simulink library "SLUGS_Library"  (Simulink 6.6)
values from neighbouring files (symbols this model uses):
  T = 0.01    [initGPS.m]    (also in mcuInit.m)
undefined symbols (not defined in the file or in its folder): apSampleTime, bankCommandLimit, daLimit, deLimit, DiscIntNeverNeededParam, drLimit, dtLimit, gaind, getWP, heightErrorLimit, mass, Ndelay, param, pitchCommandLimit, pitchErrorLimit, polesd, rollControlLimit, SampleT, Ts, u1, Xpoints, y1, yawDamperLimit, yo, Ypoints, zerosd, Zpoints
libraries: SLUGS_Library x51, simulink x32, dsPICdrivers x13, aerolibutil x2, aerolibconvert2 x1
(part 1 of 2)
settings Model: Creator=Administrator  LastModifiedBy=Elkaim

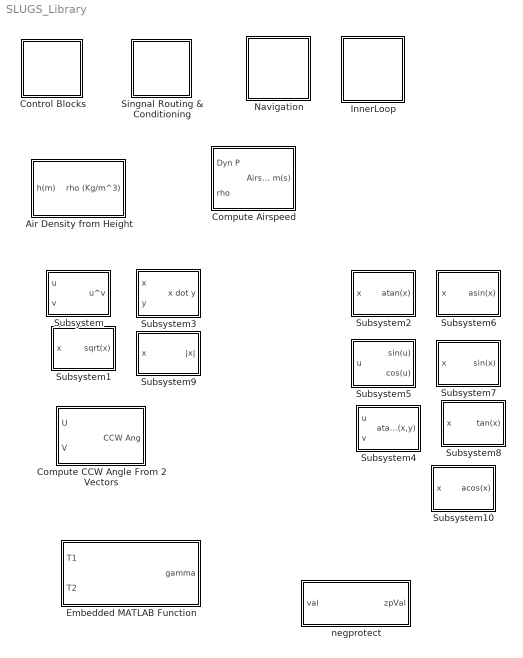
== system SLUGS_Library ==
  Air Density from Height : Subsystem  AncestorBlock=SLUGS_Library/Air Density from Height
  Compute Airspeed : Subsystem  AncestorBlock=SLUGS_Library/Compute Airspeed
  Compute CCW Angle From 2 Vectors : Subsystem
  Control Blocks : Subsystem
  Embedded MATLAB Function : Stateflow chart
  InnerLoop : Subsystem
  Navigation : Subsystem
  Singnal Routing & Conditioning : Subsystem
  Subsystem : Subsystem  AncestorBlock=SLUGS_Library/Air Density from Height/Subsystem
  Subsystem1 : Subsystem  AncestorBlock=SLUGS_Library/Compute Airspeed/Subsystem
  Subsystem10 : Subsystem
  Subsystem2 : Subsystem
  Subsystem3 : Subsystem
  Subsystem4 : Subsystem  AncestorBlock=SLUGS_Library/Air Density from Height/Subsystem
  Subsystem5 : Subsystem
  Subsystem6 : Subsystem  AncestorBlock=SLUGS_Library/Subsystem2
  Subsystem7 : Subsystem  AncestorBlock=SLUGS_Library/Subsystem2
  Subsystem8 : Subsystem
  Subsystem9 : Subsystem
  negprotect : Stateflow chart

== system SLUGS_Library/Air Density from Height ==
  h(m) : Inport
  Add : Sum  Inputs=+-  OutScaling=2^-10
  Constant : Constant  OutDataTypeMode=single
  Constant 2 from Model : Constant  Value=4.255876  OutDataTypeMode=single
  Constant from Model : Constant  Value=145442  OutDataTypeMode=single
  Divide : Product  Inputs=*/  OutScaling=2^-10
  Divide1 : Product  OutScaling=2^-10
  Length Conversion : aerolibconvert2/Length Conversion  SystemSampleTime=-1  IU=m  OU=ft
  Rho_0 (Kg/m^3) : Constant  Value=1.225  OutDataTypeMode=single
  Subsystem : SLUGS_Library/Subsystem  SystemSampleTime=-1
  rho (Kg/m^3) : Outport
  wires:
  Subsystem/1 -> Divide1/1
  Constant 2 from Model/1 -> Subsystem/2
  Add/1 -> Subsystem/1
  Length Conversion/1 -> Divide/1
  Divide1/1 -> rho (Kg/m^3)/1
  Rho_0 (Kg/m^3)/1 -> Divide1/2
  Constant from Model/1 -> Divide/2
  h(m)/1 -> Length Conversion/1
  Divide/1 -> Add/2
  Constant/1 -> Add/1

== system SLUGS_Library/Compute Airspeed ==
  Dyn P : Inport
  rho : Inport  Port=2
  Divide2 : Product  Inputs=**/  OutScaling=2^-10
  Subsystem1 : SLUGS_Library/Subsystem1  SystemSampleTime=-1
  "[ 0.01 50000]" : Saturate  UpperLimit=50000  LowerLimit=0.01
  a : Constant  Value=2  OutDataTypeMode=single
  Airspeed m(s) : Outport
  wires:
  Divide2/1 -> Subsystem1/1
  Subsystem1/1 -> Airspeed m(s)/1
  a/1 -> Divide2/1
  Dyn P/1 -> Divide2/2
  rho/1 -> "[ 0.01 50000]"/1
  "[ 0.01 50000]"/1 -> Divide2/3

== system SLUGS_Library/Compute CCW Angle From 2 Vectors ==
  U : Inport
  V : Inport  Port=2
  Add : Sum  Inputs=+-  OutScaling=2^-10
  Embedded MATLAB Function1 : Stateflow chart
  Selector : Selector  IndexOptions=Index vector (dialog)  Indices=[1]  OutputSizes=1  InputPortWidth=3
  Selector1 : Selector  IndexOptions=Index vector (dialog)  Indices=[1]  OutputSizes=1  InputPortWidth=3
  Selector2 : Selector  IndexOptions=Index vector (dialog)  Indices=[2]  OutputSizes=1  InputPortWidth=3
  Selector3 : Selector  IndexOptions=Index vector (dialog)  Indices=[2]  OutputSizes=1  InputPortWidth=3
  Subsystem1 : SLUGS_Library/Subsystem4  SystemSampleTime=-1
  Subsystem4 : SLUGS_Library/Subsystem4  SystemSampleTime=-1
  CCW Ang : Outport
  wires:
  Embedded MATLAB Function1/1(angle) -> CCW Ang/1
  V/1 -> Selector1/1, Selector2/1
  U/1 -> Selector/1, Selector3/1
  Add/1 -> Embedded MATLAB Function1/1(rawAngle)
  Subsystem1/1 -> Add/2
  Subsystem4/1 -> Add/1
  Selector1/1 -> Subsystem1/2
  Selector2/1 -> Subsystem1/1
  Selector/1 -> Subsystem4/2
  Selector3/1 -> Subsystem4/1

== system SLUGS_Library/Control Blocks ==
  PD Controller  Internal Derivative : Subsystem  mask{TSample=SampleT, NDelay=5}
      mask prompts: TSample "Sample Time"; NDelay "Derivation Time Constant Factor (1->10)"
      mask help:
      | This Block implements a PD Controller with the Following Characteristcs:
      |
      | 1.- It still expects 3 values for Gains. The second term (I) is ignored
      | 2.- The time Derivative is "low-passed" by using the previous N samples instead of the one before
  PD Controller  no Internal Derivative : Subsystem  mask{TSample=SampleT}
      mask prompts: TSample "Sample Time"
      mask help:
      | This Block implements a PD Controller with the Following Characteristcs:
      |
      | 1.- It still expects 3 values for Gains. The second term (I) is ignored
      | 2.- The time Derivative is "low-passed" by using the previous N samples instead of the one before
  PI Controller : Subsystem  mask{TSample=SampleT, upperLimit=10, lowerLimit=-10}
      mask prompts: TSample "Sample Time"; upperLimit "Integrator Upper Windup Limit"; lowerLimit "Integrator Lower Windup Limit"
      mask help:
      | This Block implements a PI Controller with the Following Characteristcs:
      |
      | 1.- Integrator antiwindup is given by the limits in the block
      | 2.-The gain still expects 3 values (the D term is ignored)
      | 3.- It contains an Integrator Reset if needed
  PID Controller : Subsystem  mask{TSample=SampleT, NDelay=5, upperLimit=10, lowerLimit=-10}
      mask prompts: TSample "Sample Time"; NDelay "Derivation Time Constant Factor (1->10)"; upperLimit "Integrator Upper Windup Limit"; lowerLimit "Integrator Lower Windup Limit"
      mask help:
      | This Block implements a PID Controller with the Following Characteristcs:
      |
      | 1.- Integrator antiwindup is given by the limits in the block
      | 2.- The time Derivative is "low-passed" by using the previous N samples instead of the one before
      | 3.- It contains an Integrator Reset if needed
  PID Controller no Internal Derivative : Subsystem  mask{TSample=SampleT, upperLimit=10, lowerLimit=-10}
      mask prompts: TSample "Sample Time"; upperLimit "Integrator Upper Windup Limit"; lowerLimit "Integrator Lower Windup Limit"
      mask help:
      | This Block implements a PID Controller with the Following Characteristcs:
      |
      | 1.- Integrator antiwindup is given by the limits in the block
      | 2.- The error time derivative is provided and therefore no derivtive block is implemented
      | 3.- It contains an Integrator Reset if needed
  PID Controller w/Anti-Windup : Subsystem  mask(PID){Tsample=Ts, Ndelay=Ndelay, SaturationLimit=deLimit}
      mask prompts: Tsample "Sample Time"; Ndelay "Integer delays for de/dt"; SaturationLimit "Saturation Limit"
      mask help: PID controller block with anti-windup and saturation limits. Implemented as a discrete forwardl integration which stops integrating when the output is saturated. Derivative is implemented as a numerical derivative with N integer delays to smooth output.
      mask Display:
      | disp('PID')
      | port_label('input',1,'error')
      | port_label('input',2,'gains')
      | port_label('output',1,'output')
  PID available Derivative w/Anti-Windup : Subsystem  mask(PID){Tsample=Ts, Ndelay=Ndelay, SaturationLimit=deLimit}
      mask prompts: Tsample "Sample Time"; Ndelay "Integer delays for de/dt"; SaturationLimit "Saturation Limit"
      mask help: PID controller block with anti-windup and saturation limits. Implemented as a discrete forwardl integration which stops integrating when the output is saturated. Derivative is implemented as a numerical derivative with N integer delays to smooth output.
      mask Display:
      | disp('PID')
      | port_label('input',1,'error')
      | port_label('input',2,'de/dt')
      | port_label('input',3,'gains')
      | port_label('output',1,'output')

== system SLUGS_Library/InnerLoop ==
  Lateral Channel : Subsystem  TreatAsAtomicUnit=on
  Longitudinal Channel : Subsystem  TreatAsAtomicUnit=on
  Navigation : Subsystem  TreatAsAtomicUnit=on

== system SLUGS_Library/Navigation ==
  Bank to Psi Dot : Subsystem
  Compute Lateral Error : Subsystem
  Compute Distance : Subsystem  AncestorBlock=SLUGS_Library/Navigation/Compute Distance
  Compute Frenet : Subsystem
  Compute WP Index : Subsystem  AncestorBlock=SLUGS_Library/Navigation/Compute WP Index
  Dot Product : simulink/Math Operations/Dot Product  InputSameDT=on  OutDataType=sfix(16)  OutScaling=2^-10  DoSatur=off
  Norm : Subsystem  AncestorBlock=SLUGS_Library/Navigation/Norm
  Normalize Vector : Subsystem
  "Park, Deyst & How Lat Accel Cmd" : Subsystem  AncestorBlock=SLUGS_Library/Navigation/Park, Deyst & How Lat Accel Cmd
  as_c to phi_c : Subsystem
  get WP Coord from Index : Subsystem  AncestorBlock=SLUGS_Library/Navigation/get WP Coord from Index
  psi_dot to Bank : Subsystem

== system SLUGS_Library/Singnal Routing & Conditioning ==
  3D Filter : Subsystem  RTWFcnName=TustinFilter3D  mask{zval=[], pval=-5, kval=5, TSample=0.01}
      mask prompts: zval "Zeros"; pval "Poles"; kval "Gains"; TSample "Sample Time"
      settings: RTWFcnNameOpts=User specified  RTWFileNameOpts=Use function name
      mask Display:
      | droots(zval,pval,kval)
      | port_label('input',1,'3D')
  3D LowPass w/Initial Condition : Subsystem  mask{a=5, yo=yo}
      mask prompts: a "Pole Location (continous)"; yo "Initial condition (3x1)"
      mask help: 3D Discrete 1st Order Low Pass filter
      mask Display:
      | port_label('input',1,'3D')
      | dpoly([a],[1 a],'s')
  Discrete Low Pass w/initial condition : Subsystem  mask{a=0.5, Yo=yo, Ts=T}
      mask prompts: a "Pole location (continuous)"; Yo "Initial condition"; Ts "Sample Time (seconds)"
      mask Display:
      | port_label('input',1,'U')
      | port_label('output',1,'Y')
      | text(0.35,0.85,'Tustin')
      | dpoly([a],[1 a],'s')
  Ellipse Correction : Subsystem  mask{param=param}
      mask prompts: param "parameter (struct)"
      mask help: Applies the correction from the ellipse algorithm to the raw data being sent through the block. The block expects a 3x1 input vector, and will return a 3x1 output vector. The parameter constant should be a struct with param.xo .yo and .zo being the offsets, param.a .b and .c being the scale factors, and param.phi .rho and .lambda being the angle non-orthogonality (in degrees).
      mask Display:
      | text(0.35,0.85,'Ellipse Correction')
      | port_label('input',1,'RAW')
      | port_label('output',1,'CORR')
  Filter : Subsystem  mask(DiscretizedZeroPole){Zeros=[], Poles=[-5], Gain=5, AbsTol=auto, SampleTime=SampleT, method=tustin, Wc=1}
      mask prompts: Zeros "Zeros (enter in s-main:)"; Poles "Poles (enter in s-domain:)"; Gain "Gain (enter in s-domain:)"; AbsTol "Absolute tolerance:"; SampleTime "Sample time:"; Wc "Critical Frequency (Hz):"
      mask help: Continuous mask uses c2d to transform parameters onto the Discrete Zero-Pole block inside.
      mask init:
      | st=SampleTime;
      | if length(st)>1
      |     st=SampleTime(1);
      | end
      | if(st>0)
      |     [zerosd,polesd,gaind] = sldiscutil('disczpk', {st,method,Wc,Zeros,Poles,Gain});
      | end	
      | s = get_param(gcb,'maskvalues');
      | zeross = s{1};
      | poless = s{2};
      | gainss = s{3};
      | %zerosc = eval(zeross);
      | %polesc = eval(poless);
      | %gainsc = eval(gainss);
      | sldiscutil('initzpkmask', st);
      | if(st==0)
      | set_param([gcb '/Zero Pole'], 'AbsoluteTolerance', AbsTol);
      | end
      mask StyleString: edit,edit,edit,edit,edit,popup(zoh|foh|tustin|prewarp|matched),edit
      mask CallbackString: |||||hidecrit|
      mask Display:
      | droots(zeross,poless,gainss)
      | text( 0.5, 1.0, method, 'verticalAlignment','top')
  Saturation : Saturate  SampleTime=SampleT
  Zero Limit : Subsystem
  myMux Fun3 : Stateflow chart

== system SLUGS_Library/Subsystem ==
  u : Inport
  v : Inport  Port=2
  C Function Call : dsPICdrivers/OTHERS/C Function Call  Tag=dsPIC_dsPIC_CFunctionCall  fctName='myPow'  INPUT_SIZE=1  INPUT1=real32  INPUT2=real32  INPUT3=--  OUTPUT_SIZE=1  OUTPUT1=real32  SampleTime=-1  InputType=[ 7 7 ]  OutputType=[ 7 ]  FctDeclaration=extern real32_T myPow(real32_T u1, real32_T u2);  FctCall=%y1 = myPow(%u1, %u2);  OrderingInOutPopup=None
  Environment Controller : simulink/Signal Routing/Environment Controller  SystemSampleTime=-1
  Math Function : Math  Operator=pow  SaturateOnIntegerOverflow=on
  u^v : Outport
  wires:
  u/1 -> C Function Call/1, Math Function/1
  v/1 -> C Function Call/2, Math Function/2
  Math Function/1 -> Environment Controller/1
  C Function Call/1 -> Environment Controller/2
  Environment Controller/1 -> u^v/1

== system SLUGS_Library/Subsystem1 ==
  x : Inport
  C Function Call : dsPICdrivers/OTHERS/C Function Call  Tag=dsPIC_dsPIC_CFunctionCall  fctName='mySqrt'  INPUT_SIZE=1  INPUT1=real32  INPUT2=--  INPUT3=--  OUTPUT_SIZE=1  OUTPUT1=real32  SampleTime=-1  InputType=[ 7 ]  OutputType=[ 7 ]  FctDeclaration=extern real32_T mySqrt(real32_T u1);  FctCall=%y1 = mySqrt(%u1);  OrderingInOutPopup=None
  Environment Controller : simulink/Signal Routing/Environment Controller  SystemSampleTime=-1
  Math Function1 : Math  Operator=sqrt  SaturateOnIntegerOverflow=on
  negprotect : Stateflow chart
  sqrt(x) : Outport
  wires:
  C Function Call/1 -> Environment Controller/2
  Math Function1/1 -> Environment Controller/1
  Environment Controller/1 -> sqrt(x)/1
  negprotect/1(zpVal) -> C Function Call/1, Math Function1/1
  x/1 -> negprotect/1(val)

== system SLUGS_Library/Subsystem10 ==
  x : Inport
  C Function Call : dsPICdrivers/OTHERS/C Function Call  Tag=dsPIC_dsPIC_CFunctionCall  fctName='myAcos'  INPUT_SIZE=1  INPUT1=real32  INPUT2=--  INPUT3=--  OUTPUT_SIZE=1  OUTPUT1=real32  SampleTime=-1  InputType=[ 7 ]  OutputType=[ 7 ]  FctDeclaration=extern real32_T myAcos(real32_T u1);  FctCall=%y1 = myAcos(%u1);  OrderingInOutPopup=None
  Environment Controller : simulink/Signal Routing/Environment Controller  SystemSampleTime=-1
  Trigonometric Function : Trigonometry  Operator=acos
  acos(x) : Outport
  wires:
  x/1 -> C Function Call/1, Trigonometric Function/1
  Trigonometric Function/1 -> Environment Controller/1
  C Function Call/1 -> Environment Controller/2
  Environment Controller/1 -> acos(x)/1

== system SLUGS_Library/Subsystem2 ==
  x : Inport
  C Function Call : dsPICdrivers/OTHERS/C Function Call  Tag=dsPIC_dsPIC_CFunctionCall  fctName='myAtan'  INPUT_SIZE=1  INPUT1=real32  INPUT2=--  INPUT3=--  OUTPUT_SIZE=1  OUTPUT1=real32  SampleTime=-1  InputType=[ 7 ]  OutputType=[ 7 ]  FctDeclaration=extern real32_T myAtan(real32_T u1);  FctCall=%y1 = myAtan(%u1);  OrderingInOutPopup=None
  Environment Controller : simulink/Signal Routing/Environment Controller  SystemSampleTime=-1
  Trigonometric Function : Trigonometry  Operator=atan
  atan(x) : Outport
  wires:
  Environment Controller/1 -> atan(x)/1
  C Function Call/1 -> Environment Controller/2
  Trigonometric Function/1 -> Environment Controller/1
  x/1 -> Trigonometric Function/1, C Function Call/1

== system SLUGS_Library/Subsystem3 ==
  x : Inport
  y : Inport  Port=2
  Dot Product : simulink/Math Operations/Dot Product  InputSameDT=on  OutDataType=sfix(16)  OutScaling=2^-10  DoSatur=off
  Embedded MATLAB Function : Stateflow chart
  Environment Controller : simulink/Signal Routing/Environment Controller  SystemSampleTime=-1
  x dot y : Outport
  wires:
  y/1 -> Embedded MATLAB Function/2(y), Dot Product/2
  x/1 -> Embedded MATLAB Function/1(x), Dot Product/1
  Dot Product/1 -> Environment Controller/1
  Embedded MATLAB Function/1(xDoty) -> Environment Controller/2
  Environment Controller/1 -> x dot y/1

== system SLUGS_Library/Subsystem4 ==
  u : Inport
  v : Inport  Port=2
  C Function Call : dsPICdrivers/OTHERS/C Function Call  Tag=dsPIC_dsPIC_CFunctionCall  fctName='myAtan2'  INPUT_SIZE=1  INPUT1=real32  INPUT2=real32  INPUT3=--  OUTPUT_SIZE=1  OUTPUT1=real32  SampleTime=-1  InputType=[ 7 7 ]  OutputType=[ 7 ]  FctDeclaration=extern real32_T myAtan2(real32_T u1, real32_T u2);  FctCall=%y1 = myAtan2(%u1, %u2);  OrderingInOutPopup=None
  Environment Controller : simulink/Signal Routing/Environment Controller  SystemSampleTime=-1
  Trigonometric Function : Trigonometry  Operator=atan2
  atan2(x,y) : Outport
  wires:
  u/1 -> Trigonometric Function/1, C Function Call/1
  v/1 -> Trigonometric Function/2, C Function Call/2
  Trigonometric Function/1 -> Environment Controller/1
  C Function Call/1 -> Environment Controller/2
  Environment Controller/1 -> atan2(x,y)/1

== system SLUGS_Library/Subsystem5 ==
  u : Inport
  C Function Call : dsPICdrivers/OTHERS/C Function Call  Tag=dsPIC_dsPIC_CFunctionCall  fctName='mySin'  INPUT_SIZE=1  INPUT1=real32  INPUT2=--  INPUT3=--  OUTPUT_SIZE=1  OUTPUT1=real32  SampleTime=-1  InputType=[ 7 ]  OutputType=[ 7 ]  FctDeclaration=extern real32_T mySin(real32_T u1);  FctCall=%y1 = mySin(%u1);  OrderingInOutPopup=None
  C Function Call1 : dsPICdrivers/OTHERS/C Function Call  Tag=dsPIC_dsPIC_CFunctionCall  fctName='myCos'  INPUT_SIZE=1  INPUT1=real32  INPUT2=--  INPUT3=--  OUTPUT_SIZE=1  OUTPUT1=real32  SampleTime=-1  InputType=[ 7 ]  OutputType=[ 7 ]  FctDeclaration=extern real32_T myCos(real32_T u1);  FctCall=%y1 = myCos(%u1);  OrderingInOutPopup=None
  Environment Controller : simulink/Signal Routing/Environment Controller  SystemSampleTime=-1
  Environment Controller1 : simulink/Signal Routing/Environment Controller  SystemSampleTime=-1
  SinCos1 : aerolibutil/SinCos  SystemSampleTime=-1
  sin(u) : Outport
  cos(u) : Outport  Port=2
  wires:
  SinCos1/2 -> Environment Controller1/1
  C Function Call1/1 -> Environment Controller1/2
  Environment Controller1/1 -> cos(u)/1
  u/1 -> C Function Call1/1, C Function Call/1, SinCos1/1
  SinCos1/1 -> Environment Controller/1
  C Function Call/1 -> Environment Controller/2
  Environment Controller/1 -> sin(u)/1

== system SLUGS_Library/Subsystem6 ==
  x : Inport
  C Function Call : dsPICdrivers/OTHERS/C Function Call  Tag=dsPIC_dsPIC_CFunctionCall  fctName='myAsin'  INPUT_SIZE=1  INPUT1=real32  INPUT2=--  INPUT3=--  OUTPUT_SIZE=1  OUTPUT1=real32  SampleTime=-1  InputType=[ 7 ]  OutputType=[ 7 ]  FctDeclaration=extern real32_T myAsin(real32_T u1);  FctCall=%y1 = myAsin(%u1);  OrderingInOutPopup=None
  Environment Controller : simulink/Signal Routing/Environment Controller  SystemSampleTime=-1
  Trigonometric Function : Trigonometry  Operator=asin
  "[-1,1]" : Saturate  UpperLimit=0.9999  LowerLimit=-0.999
  asin(x) : Outport
  wires:
  Environment Controller/1 -> asin(x)/1
  C Function Call/1 -> Environment Controller/2
  Trigonometric Function/1 -> Environment Controller/1
  x/1 -> "[-1,1]"/1
  "[-1,1]"/1 -> Trigonometric Function/1, C Function Call/1

== system SLUGS_Library/Subsystem7 ==
  x : Inport
  C Function Call : dsPICdrivers/OTHERS/C Function Call  Tag=dsPIC_dsPIC_CFunctionCall  fctName='mySin'  INPUT_SIZE=1  INPUT1=real32  INPUT2=--  INPUT3=--  OUTPUT_SIZE=1  OUTPUT1=real32  SampleTime=-1  InputType=[ 7 ]  OutputType=[ 7 ]  FctDeclaration=extern real32_T mySin(real32_T u1);  FctCall=%y1 = mySin(%u1);  OrderingInOutPopup=None
  Environment Controller : simulink/Signal Routing/Environment Controller  SystemSampleTime=-1
  Trigonometric Function : Trigonometry
  sin(x) : Outport
  wires:
  Environment Controller/1 -> sin(x)/1
  C Function Call/1 -> Environment Controller/2
  Trigonometric Function/1 -> Environment Controller/1
  x/1 -> Trigonometric Function/1, C Function Call/1

== system SLUGS_Library/Subsystem8 ==
  x : Inport
  C Function Call : dsPICdrivers/OTHERS/C Function Call  Tag=dsPIC_dsPIC_CFunctionCall  fctName='myTan'  INPUT_SIZE=1  INPUT1=real32  INPUT2=--  INPUT3=--  OUTPUT_SIZE=1  OUTPUT1=real32  SampleTime=-1  InputType=[ 7 ]  OutputType=[ 7 ]  FctDeclaration=extern real32_T myTan(real32_T u1);  FctCall=%y1 = myTan(%u1);  OrderingInOutPopup=None
  Environment Controller : simulink/Signal Routing/Environment Controller  SystemSampleTime=-1
  Trigonometric Function : Trigonometry  Operator=tan
  tan(x) : Outport
  wires:
  x/1 -> C Function Call/1, Trigonometric Function/1
  Trigonometric Function/1 -> Environment Controller/1
  C Function Call/1 -> Environment Controller/2
  Environment Controller/1 -> tan(x)/1

== system SLUGS_Library/Subsystem9 ==
  x : Inport
  Abs : Abs
  C Function Call : dsPICdrivers/OTHERS/C Function Call  Tag=dsPIC_dsPIC_CFunctionCall  fctName='myAbs'  INPUT_SIZE=1  INPUT1=real32  INPUT2=--  INPUT3=--  OUTPUT_SIZE=1  OUTPUT1=real32  SampleTime=-1  InputType=[ 7 ]  OutputType=[ 7 ]  FctDeclaration=extern real32_T myAbs(real32_T u1);  FctCall=%y1 = myAbs(%u1);  OrderingInOutPopup=None
  Environment Controller : simulink/Signal Routing/Environment Controller  SystemSampleTime=-1
  |x| : Outport
  wires:
  x/1 -> Abs/1, C Function Call/1
  C Function Call/1 -> Environment Controller/2
  Abs/1 -> Environment Controller/1
  Environment Controller/1 -> |x|/1

== system SLUGS_Library/Control Blocks/PD Controller  Internal Derivative ==
  note: This Block implements a PID Controller with the
      | Following Characteristcs:
      | 1.- Antiwindup is given by the Limits in the block
      | 2.- The time Derivative is "low-passed" by using the
      | previous N samples instead of the one before
      | 3.- It contains an Integrator Reset if needed
  Error : Inport
  PID Gains : Inport  Port=2
  Add : Sum  Inputs=2  OutScaling=2^-10
  Demux : Demux  Outputs=3
  Divide : Product  OutScaling=2^-10
  Divide2 : Product  OutScaling=2^-10
  Low_passed Time Derivative : Subsystem
  Terminator : Terminator
  Control : Outport
  wires:
  Divide2/1 -> Add/2
  Demux/3 -> Divide2/1
  Add/1 -> Control/1
  Divide/1 -> Add/1
  Demux/1 -> Divide/1
  PID Gains/1 -> Demux/1
  Error/1 -> Low_passed Time Derivative/1(f(t)), Divide/2
  Low_passed Time Derivative/1(f_dot(t)) -> Divide2/2
  Demux/2 -> Terminator/1

== system SLUGS_Library/Control Blocks/PD Controller  no Internal Derivative ==
  note: This Block implements a PID Controller with the
      | Following Characteristcs:
      | 1.- Antiwindup is given by the Limits in the block
      | 2.-No time derivative
      | 3.- It contains an Integrator Reset if needed
  Error : Inport
  Error Dot : Inport  Port=2
  PID Gains : Inport  Port=3
  Add : Sum  Inputs=2  OutScaling=2^-10
  Demux : Demux  Outputs=3
  Divide : Product  OutScaling=2^-10
  Divide2 : Product  OutScaling=2^-10
  Terminator : Terminator
  Control : Outport
  wires:
  Demux/2 -> Terminator/1
  Error Dot/1 -> Divide2/2
  Error/1 -> Divide/2
  PID Gains/1 -> Demux/1
  Demux/1 -> Divide/1
  Divide/1 -> Add/1
  Add/1 -> Control/1
  Demux/3 -> Divide2/1
  Divide2/1 -> Add/2

== system SLUGS_Library/Control Blocks/PI Controller ==
  note: This Block implements a PID Controller with the
      | Following Characteristcs:
      | 1.- Antiwindup is given by the Limits in the block
      | 2.- The error derivative is provided and therefore no
      | time derivative is implemented
      | 3.- It contains an Integrator Reset if needed
  Error : Inport
  Int Reset : Inport  Port=2
  Int IC : Inport  Port=3
  PID Gains : Inport  Port=4
  Add : Sum  Inputs=2  OutDataTypeMode=single  OutScaling=2^-10
  Demux : Demux  Outputs=3
  Discrete-Time Integrator : DiscreteIntegrator  IntegratorMethod=Integration: Trapezoidal  ExternalReset=sampled level  InitialConditionSource=external  SampleTime=TSample  OutDataTypeMode=single  LimitOutput=on  UpperSaturationLimit=upperLimit  LowerSaturationLimit=lowerLimit  ICPrevOutput=DiscIntNeverNeededParam  ICPrevScaledInput=DiscIntNeverNeededParam
  Divide : Product  OutDataTypeMode=single  OutScaling=2^-10
  Divide1 : Product  OutDataTypeMode=single  OutScaling=2^-10
  Terminator : Terminator
  Control : Outport
  wires:
  Error/1 -> Discrete-Time Integrator/1, Divide/2
  Int Reset/1 -> Discrete-Time Integrator/2
  Discrete-Time Integrator/1 -> Divide1/2
  Int IC/1 -> Discrete-Time Integrator/3
  PID Gains/1 -> Demux/1
  Demux/1 -> Divide/1
  Divide/1 -> Add/1
  Add/1 -> Control/1
  Demux/2 -> Divide1/1
  Divide1/1 -> Add/2
  Demux/3 -> Terminator/1

== system SLUGS_Library/Control Blocks/PID Controller ==
  note: This Block implements a PID Controller with the
      | Following Characteristcs:
      | 1.- Antiwindup is given by the Limits in the block
      | 2.- The time Derivative is "low-passed" by using the
      | previous N samples instead of the one before
      | 3.- It contains an Integrator Reset if needed
  Error : Inport
  Int Reset : Inport  Port=2
  Int IC : Inport  Port=3
  PID Gains : Inport  Port=4
  Add : Sum  Inputs=3  OutScaling=2^-10
  Demux : Demux  Outputs=3
  Discrete-Time Integrator : DiscreteIntegrator  IntegratorMethod=Integration: Trapezoidal  ExternalReset=sampled level  InitialConditionSource=external  SampleTime=TSample  OutDataTypeMode=single  LimitOutput=on  UpperSaturationLimit=upperLimit  LowerSaturationLimit=lowerLimit  ICPrevOutput=DiscIntNeverNeededParam  ICPrevScaledInput=DiscIntNeverNeededParam
  Divide : Product  OutScaling=2^-10
  Divide1 : Product  OutScaling=2^-10
  Divide2 : Product  OutScaling=2^-10
  Low_passed Time Derivative : Subsystem
  Control : Outport
  wires:
  Low_passed Time Derivative/1(f_dot(t)) -> Divide2/2
  Error/1 -> Discrete-Time Integrator/1, Divide/2, Low_passed Time Derivative/1(f(t))
  Int Reset/1 -> Discrete-Time Integrator/2
  Discrete-Time Integrator/1 -> Divide1/2
  Int IC/1 -> Discrete-Time Integrator/3
  PID Gains/1 -> Demux/1
  Demux/1 -> Divide/1
  Divide/1 -> Add/1
  Add/1 -> Control/1
  Demux/2 -> Divide1/1
  Demux/3 -> Divide2/1
  Divide1/1 -> Add/2
  Divide2/1 -> Add/3

== system SLUGS_Library/Control Blocks/PID Controller no Internal Derivative ==
  note: This Block implements a PID Controller with the
      | Following Characteristcs:
      | 1.- Antiwindup is given by the Limits in the block
      | 2.- The error derivative is provided and therefore no
      | time derivative is implemented
      | 3.- It contains an Integrator Reset if needed
  Error : Inport
  Error dot : Inport  Port=2
  Int Reset : Inport  Port=3
  Int IC : Inport  Port=4
  PID Gains : Inport  Port=5
  Add : Sum  Inputs=3  OutScaling=2^-10
  Demux : Demux  Outputs=3
  Discrete-Time Integrator : DiscreteIntegrator  IntegratorMethod=Integration: Trapezoidal  ExternalReset=sampled level  InitialConditionSource=external  SampleTime=TSample  LimitOutput=on  UpperSaturationLimit=upperLimit  LowerSaturationLimit=lowerLimit  ICPrevOutput=DiscIntNeverNeededParam  ICPrevScaledInput=DiscIntNeverNeededParam
  Divide : Product  OutScaling=2^-10
  Divide1 : Product  OutScaling=2^-10
  Divide2 : Product  OutScaling=2^-10
  Control : Outport
  wires:
  Divide2/1 -> Add/3
  Divide1/1 -> Add/2
  Demux/3 -> Divide2/1
  Demux/2 -> Divide1/1
  Add/1 -> Control/1
  Divide/1 -> Add/1
  Demux/1 -> Divide/1
  PID Gains/1 -> Demux/1
  Int IC/1 -> Discrete-Time Integrator/3
  Discrete-Time Integrator/1 -> Divide1/2
  Int Reset/1 -> Discrete-Time Integrator/2
  Error/1 -> Divide/2, Discrete-Time Integrator/1
  Error dot/1 -> Divide2/2

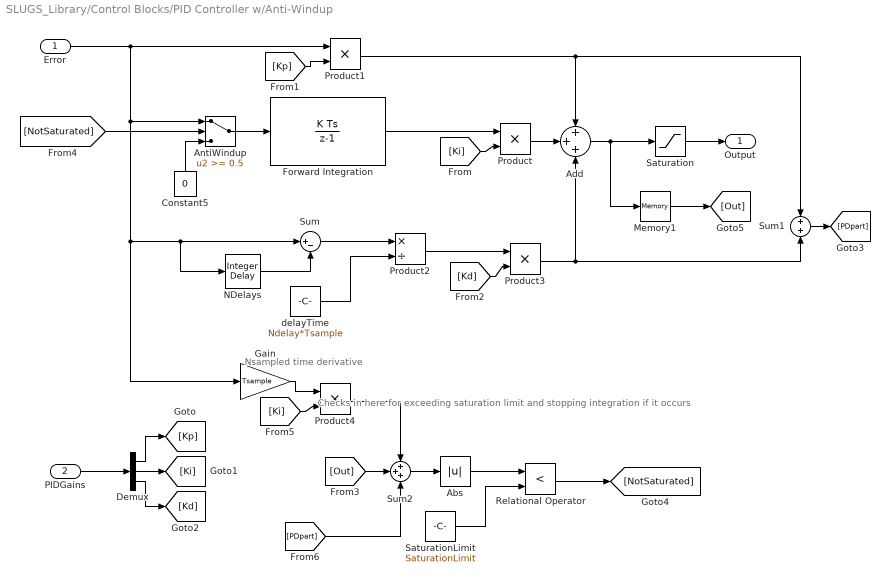
== system SLUGS_Library/Control Blocks/PID Controller w/Anti-Windup ==
  note: Nsampled time derivative
  note: Checks in here for
      | exceeding saturation
      | limit and stopping
      | integration if it occurs
  Error : Inport
  PIDGains : Inport  Port=2
  Abs : Abs
  Add : Sum  Inputs=+++  OutScaling=2^-10
  AntiWindup : Switch  Threshold=0.5
  Constant5 : Constant  Orientation=up  Value=0  OutDataTypeMode=double
  Demux : Demux  Outputs=3
  Forward Integration : DiscreteIntegrator  SampleTime=Tsample  ICPrevOutput=DiscIntNeverNeededParam  ICPrevScaledInput=DiscIntNeverNeededParam
  Gain : Gain  Gain=Tsample
  Memory1 : Memory  InheritSampleTime=on
  NDelays : simulink/Discrete/Integer Delay  vinit=0.0  samptime=Tsample  NumDelays=Ndelay
  Product{,1,3..4} (4 alike) : Product  RndMeth=Zero
  Product2 : Product  Inputs=*/  RndMeth=Zero
  Relational Operator : RelationalOperator  Operator=<  LogicOutDataTypeMode=Boolean
  Saturation : Saturate  UpperLimit=SaturationLimit  LowerLimit=-SaturationLimit
  SaturationLimit : Constant  Value=SaturationLimit
  Sum : Sum  Inputs=|+-
  Sum1 : Sum  Inputs=+|+
  Sum2 : Sum  Inputs=+++
  delayTime : Constant  Value=Ndelay*Tsample
  Output : Outport
  wires:
  [NotSaturated] -> AntiWindup/2
  Abs/1 -> Relational Operator/1
  SaturationLimit/1 -> Relational Operator/2
  Saturation/1 -> Output/1
  Product3/1 -> Add/3, Sum1/2
  Product2/1 -> Product3/1
  [Kd] -> Product3/2
  delayTime/1 -> Product2/2
  Sum/1 -> Product2/1
  NDelays/1 -> Sum/2
  Add/1 -> Saturation/1, Memory1/1
  Product1/1 -> Sum1/1, Add/1
  Product/1 -> Add/2
  [Kp] -> Product1/2
  Forward Integration/1 -> Product/1
  [Ki] -> Product/2
  Error/1 -> Product1/1, AntiWindup/1, Gain/1, Sum/1, NDelays/1
  AntiWindup/1 -> Forward Integration/1
  Constant5/1 -> AntiWindup/3
  Demux/3 -> [Kd]
  Demux/2 -> [Ki]
  Demux/1 -> [Kp]
  PIDGains/1 -> Demux/1
  Sum1/1 -> [PDpart]
  [Out] -> Sum2/2
  Sum2/1 -> Abs/1
  [Ki] -> Product4/2
  Gain/1 -> Product4/1
  Product4/1 -> Sum2/1
  Memory1/1 -> [Out]
  [PDpart] -> Sum2/3
  Relational Operator/1 -> [NotSaturated]

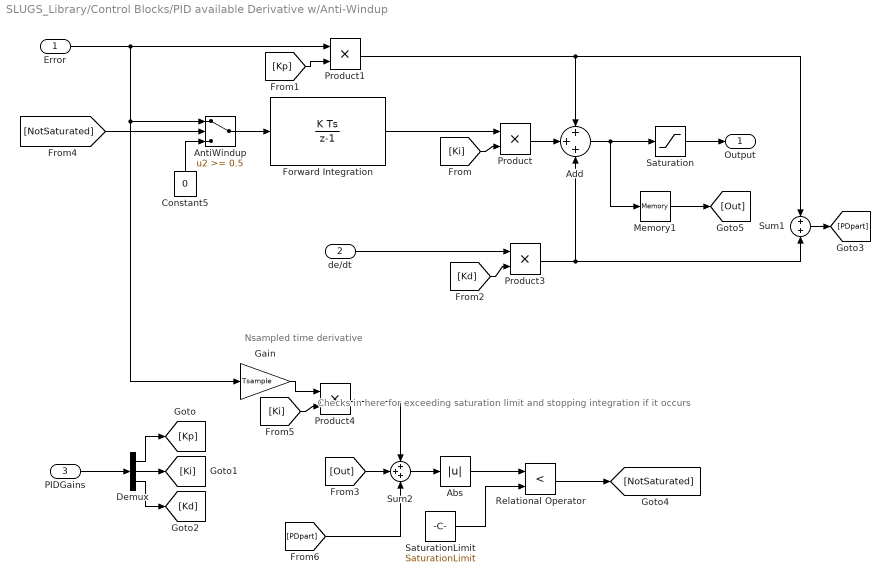
== system SLUGS_Library/Control Blocks/PID available Derivative w/Anti-Windup ==
  note: Checks in here for
      | exceeding saturation
      | limit and stopping
      | integration if it occurs
  note: Nsampled time derivative
  Error : Inport
  de/dt : Inport  Port=2
  PIDGains : Inport  Port=3
  Abs : Abs
  Add : Sum  Inputs=+++  OutScaling=2^-10
  AntiWindup : Switch  Threshold=0.5
  Constant5 : Constant  Orientation=up  Value=0  OutDataTypeMode=double
  Demux : Demux  Outputs=3
  Forward Integration : DiscreteIntegrator  SampleTime=Tsample  ICPrevOutput=DiscIntNeverNeededParam  ICPrevScaledInput=DiscIntNeverNeededParam
  Gain : Gain  Gain=Tsample
  Memory1 : Memory  InheritSampleTime=on
  Product{,1,3..4} (4 alike) : Product  RndMeth=Zero
  Relational Operator : RelationalOperator  Operator=<  LogicOutDataTypeMode=Boolean
  Saturation : Saturate  UpperLimit=SaturationLimit  LowerLimit=-SaturationLimit
  SaturationLimit : Constant  Value=SaturationLimit
  Sum1 : Sum  Inputs=+|+
  Sum2 : Sum  Inputs=+++
  Output : Outport
  wires:
  Relational Operator/1 -> [NotSaturated]
  [PDpart] -> Sum2/3
  Memory1/1 -> [Out]
  Product4/1 -> Sum2/1
  Gain/1 -> Product4/1
  [Ki] -> Product4/2
  Sum2/1 -> Abs/1
  [Out] -> Sum2/2
  Sum1/1 -> [PDpart]
  PIDGains/1 -> Demux/1
  Demux/1 -> [Kp]
  Demux/2 -> [Ki]
  Demux/3 -> [Kd]
  Constant5/1 -> AntiWindup/3
  AntiWindup/1 -> Forward Integration/1
  Error/1 -> Gain/1, AntiWindup/1, Product1/1
  [Ki] -> Product/2
  Forward Integration/1 -> Product/1
  [Kp] -> Product1/2
  Product/1 -> Add/2
  Product1/1 -> Add/1, Sum1/1
  Add/1 -> Memory1/1, Saturation/1
  [Kd] -> Product3/2
  de/dt/1 -> Product3/1
  Product3/1 -> Sum1/2, Add/3
  Saturation/1 -> Output/1
  SaturationLimit/1 -> Relational Operator/2
  Abs/1 -> Relational Operator/1
  [NotSaturated] -> AntiWindup/2

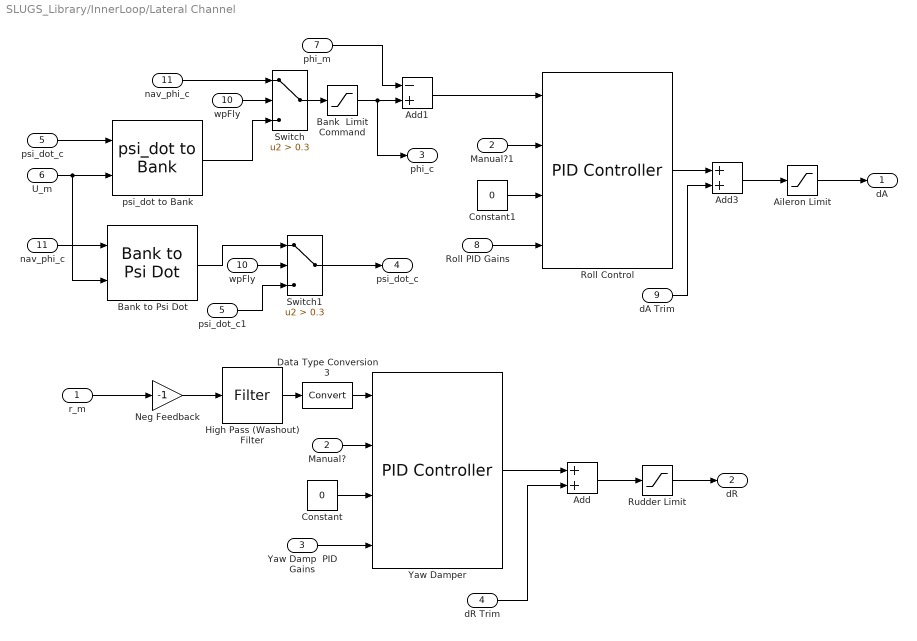
== system SLUGS_Library/InnerLoop/Lateral Channel ==
  r_m : Inport
  Manual? : Inport  Port=2
  Yaw Damp  PID Gains : Inport  Port=3
  dR Trim : Inport  Port=4
  psi_dot_c : Inport  Port=5
  U_m : Inport  Port=6
  phi_m : Inport  Port=7
  Roll PID Gains : Inport  Port=8
  dA Trim : Inport  Port=9
  wpFly : Inport  Port=10  SampleTime=apSampleTime
  nav_phi_c : Inport  Port=11
  Add : Sum  OutDataTypeMode=single  OutScaling=2^-10
  Add1 : Sum  Inputs=-+  OutDataTypeMode=single  OutScaling=2^-10
  Add3 : Sum  OutDataTypeMode=single  OutScaling=2^-10
  Aileron Limit : Saturate  UpperLimit=daLimit  LowerLimit=-daLimit  SampleTime=apSampleTime
  Bank  Limit Command : Saturate  UpperLimit=bankCommandLimit  LowerLimit=-bankCommandLimit  SampleTime=apSampleTime
  Bank to Psi Dot : SLUGS_Library/Navigation/Bank to Psi Dot  SystemSampleTime=-1
  Constant : Constant  Value=0  OutDataTypeMode=single
  Constant1 : Constant  Value=0  OutDataTypeMode=single
  Data Type Conversion3 : DataTypeConversion  OutDataTypeMode=single
  High Pass (Washout) Filter : SLUGS_Library/Singnal Routing & Conditioning/Filter  SystemSampleTime=-1  Zeros=[0]  Poles=[-1/5]  Gain=1  AbsTol=auto  SampleTime=apSampleTime  method=tustin  Wc=1
  Manual?1 : InportShadow  Port=2  LatchByCopyingInsideSignal=off
  Neg Feedback : Gain  Gain=-1  OutDataTypeMode=Specify via dialog  OutDataType=float('double')
  Roll Control : SLUGS_Library/Control Blocks/PID Controller  SystemSampleTime=-1  TSample=apSampleTime  NDelay=derivativesConstant  upperLimit=rollControlLimit  lowerLimit=-rollControlLimit
  Rudder Limit : Saturate  UpperLimit=apSampleTime  LowerLimit=-drLimit  SampleTime=apSampleTime
  Switch : Switch  Criteria=u2 > Threshold  Threshold=0.3
  Switch1 : Switch  Criteria=u2 > Threshold  Threshold=0.3  InputSameDT=on
  Yaw Damper : SLUGS_Library/Control Blocks/PID Controller  SystemSampleTime=-1  TSample=apSampleTime  NDelay=derivativesConstant  upperLimit=yawDamperLimit  lowerLimit=-yawDamperLimit
  "nav_phi_c  " : InportShadow  Port=11  LatchByCopyingInsideSignal=off
  psi_dot to Bank : SLUGS_Library/Navigation/psi_dot to Bank  SystemSampleTime=-1
  psi_dot_c1 : InportShadow  Port=5  LatchByCopyingInsideSignal=off
  "wpFly " : InportShadow  Port=10  SampleTime=apSampleTime  LatchByCopyingInsideSignal=off
  dA : Outport
  dR : Outport  Port=2
  phi_c : Outport  Port=3
  "psi_dot_c " : Outport  Port=4
  wires:
  High Pass (Washout) Filter/1 -> Data Type Conversion3/1
  Neg Feedback/1 -> High Pass (Washout) Filter/1
  r_m/1 -> Neg Feedback/1
  Rudder Limit/1 -> dR/1
  Constant/1 -> Yaw Damper/3
  Manual?/1 -> Yaw Damper/2
  Yaw Damp  PID Gains/1 -> Yaw Damper/4
  Add/1 -> Rudder Limit/1
  Yaw Damper/1 -> Add/1
  dR Trim/1 -> Add/2
  psi_dot_c/1 -> psi_dot to Bank/1
  U_m/1 -> Bank to Psi Dot/2, psi_dot to Bank/2
  Manual?1/1 -> Roll Control/2
  Constant1/1 -> Roll Control/3
  Roll PID Gains/1 -> Roll Control/4
  Add3/1 -> Aileron Limit/1
  Roll Control/1 -> Add3/1
  dA Trim/1 -> Add3/2
  Aileron Limit/1 -> dA/1
  Add1/1 -> Roll Control/1
  phi_m/1 -> Add1/1
  Switch/1 -> Bank  Limit Command/1
  nav_phi_c/1 -> Switch/1
  wpFly/1 -> Switch/2
  psi_dot to Bank/1 -> Switch/3
  Bank  Limit Command/1 -> Add1/2, phi_c/1
  "wpFly "/1 -> Switch1/2
  Switch1/1 -> "psi_dot_c "/1
  "nav_phi_c  "/1 -> Bank to Psi Dot/1
  Bank to Psi Dot/1 -> Switch1/1
  psi_dot_c1/1 -> Switch1/3
  Data Type Conversion3/1 -> Yaw Damper/1

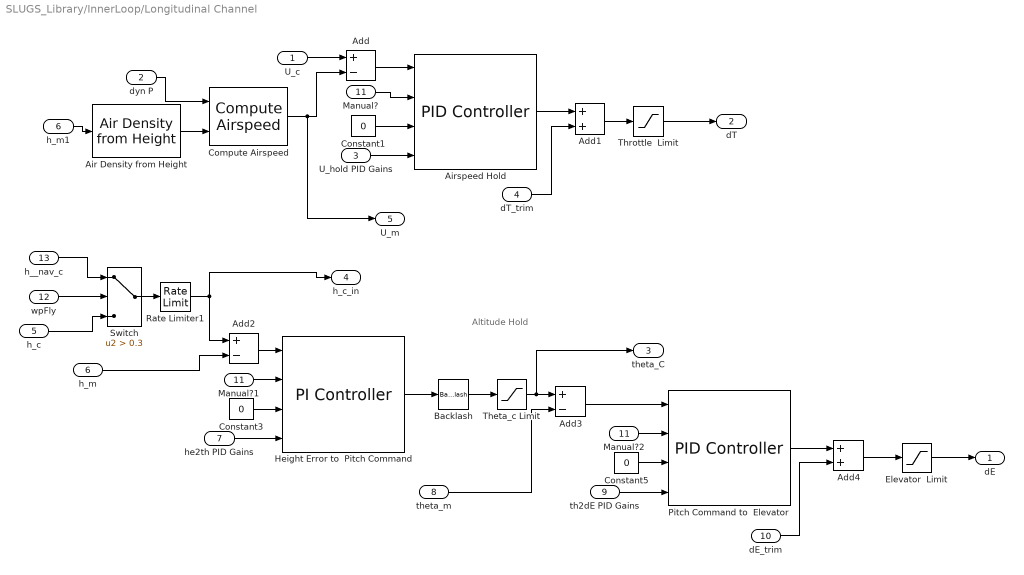
== system SLUGS_Library/InnerLoop/Longitudinal Channel ==
  note: Altitude Hold
  U_c : Inport
  dyn P : Inport  Port=2
  U_hold PID Gains : Inport  Port=3
  dT_trim : Inport  Port=4
  h_c : Inport  Port=5
  h_m : Inport  Port=6
  he2th PID Gains : Inport  Port=7
  theta_m : Inport  Port=8
  th2dE PID Gains : Inport  Port=9
  dE_trim : Inport  Port=10
  Manual? : Inport  Port=11
  wpFly : Inport  Port=12  SampleTime=apSampleTime
  h__nav_c : Inport  Port=13
  Add : Sum  Inputs=+-  OutScaling=2^-10
  Add1 : Sum  Inputs=2  OutDataTypeMode=single  OutScaling=2^-10
  Add2 : Sum  Inputs=+-  OutDataTypeMode=single  OutScaling=2^-10
  Add3 : Sum  Inputs=+-  OutDataTypeMode=single  OutScaling=2^-10
  Add4 : Sum  Inputs=2  OutDataTypeMode=single  OutScaling=2^-10
  Air Density from Height : SLUGS_Library/Air Density from Height  SystemSampleTime=-1
  Airspeed Hold : SLUGS_Library/Control Blocks/PID Controller  SystemSampleTime=-1  TSample=apSampleTime  NDelay=derivativesConstant  upperLimit=uHoldLimit  lowerLimit=0.1
  Backlash : Backlash  BacklashWidth=0.05
  Compute Airspeed : SLUGS_Library/Compute Airspeed  SystemSampleTime=-1
  Constant1 : Constant  Value=0  OutDataTypeMode=single
  Constant3 : Constant  Value=0  OutDataTypeMode=single
  Constant5 : Constant  Value=0  OutDataTypeMode=single
  Elevator  Limit : Saturate  UpperLimit=deLimit  LowerLimit=-deLimit  SampleTime=apSampleTime
  Height Error to  Pitch Command : SLUGS_Library/Control Blocks/PI Controller  SystemSampleTime=-1  TSample=apSampleTime  upperLimit=heightErrorLimit  lowerLimit=-heightErrorLimit
  Manual?1 : InportShadow  Port=11  LatchByCopyingInsideSignal=off
  Manual?2 : InportShadow  Port=11  LatchByCopyingInsideSignal=off
  Pitch Command to  Elevator : SLUGS_Library/Control Blocks/PID Controller  SystemSampleTime=-1  TSample=apSampleTime  NDelay=derivativesConstant  upperLimit=pitchErrorLimit  lowerLimit=-pitchErrorLimit
  Rate Limiter1 : RateLimiter  RisingSlewLimit=10  FallingSlewLimit=-10  SampleTimeMode=inherited
  Switch : Switch  Criteria=u2 > Threshold  Threshold=0.3  InputSameDT=on
  Theta_c Limit : Saturate  UpperLimit=pitchCommandLimit  LowerLimit=-pitchCommandLimit  SampleTime=apSampleTime
  Throttle  Limit : Saturate  UpperLimit=dtLimit  LowerLimit=0  SampleTime=apSampleTime
  h_m1 : InportShadow  Port=6  LatchByCopyingInsideSignal=off
  dE : Outport
  dT : Outport  Port=2
  theta_C : Outport  Port=3
  h_c_in : Outport  Port=4
  U_m : Outport  Port=5
  wires:
  U_c/1 -> Add/1
  Compute Airspeed/1 -> Add/2, U_m/1
  Add/1 -> Airspeed Hold/1
  Airspeed Hold/1 -> Add1/1
  dT_trim/1 -> Add1/2
  Add1/1 -> Throttle  Limit/1
  Constant1/1 -> Airspeed Hold/3
  U_hold PID Gains/1 -> Airspeed Hold/4
  Throttle  Limit/1 -> dT/1
  Add2/1 -> Height Error to  Pitch Command/1
  h_m/1 -> Add2/2
  Constant3/1 -> Height Error to  Pitch Command/3
  theta_m/1 -> Add3/2
  Constant5/1 -> Pitch Command to  Elevator/3
  Manual?/1 -> Airspeed Hold/2
  Manual?1/1 -> Height Error to  Pitch Command/2
  Manual?2/1 -> Pitch Command to  Elevator/2
  Add4/1 -> Elevator  Limit/1
  Pitch Command to  Elevator/1 -> Add4/1
  dE_trim/1 -> Add4/2
  Elevator  Limit/1 -> dE/1
  Air Density from Height/1 -> Compute Airspeed/2
  dyn P/1 -> Compute Airspeed/1
  h_m1/1 -> Air Density from Height/1
  he2th PID Gains/1 -> Height Error to  Pitch Command/4
  th2dE PID Gains/1 -> Pitch Command to  Elevator/4
  Add3/1 -> Pitch Command to  Elevator/1
  Theta_c Limit/1 -> Add3/1, theta_C/1
  wpFly/1 -> Switch/2
  Switch/1 -> Rate Limiter1/1
  h_c/1 -> Switch/3
  h__nav_c/1 -> Switch/1
  Rate Limiter1/1 -> Add2/1, h_c_in/1
  Height Error to  Pitch Command/1 -> Backlash/1
  Backlash/1 -> Theta_c Limit/1

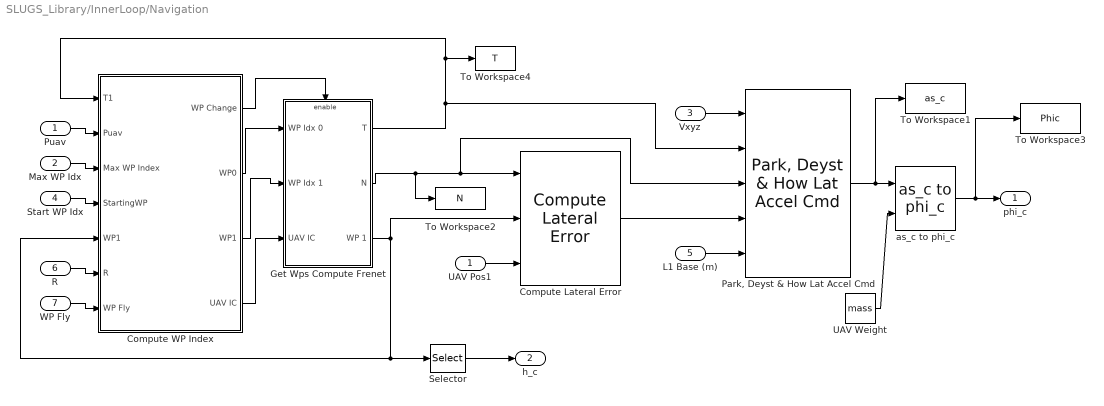
== system SLUGS_Library/InnerLoop/Navigation ==
  Puav : Inport  SampleTime=apSampleTime
  Max WP Idx : Inport  Port=2
  Vxyz : Inport  Port=3
  Start WP Idx : Inport  Port=4
  L1 Base (m) : Inport  Port=5
  R : Inport  Port=6
  WP Fly : Inport  Port=7
  Compute Lateral Error : SLUGS_Library/Navigation/Compute Lateral Error  SystemSampleTime=-1
  Compute WP Index : Subsystem  AncestorBlock=SLUGS_Library/Navigation/Compute WP Index
  Get Wps Compute Frenet : Subsystem
  "Park, Deyst & How Lat Accel Cmd" : SLUGS_Library/Navigation/Park, Deyst & How Lat Accel Cmd  SystemSampleTime=-1
  Selector : Selector  IndexOptions=Index vector (dialog)  Indices=[3]  OutputSizes=1  InputPortWidth=3
  To Workspace1 : ToWorkspace  VariableName=as_c  SampleTime=-1  SaveFormat=Array
  To Workspace2 : ToWorkspace  VariableName=N  SampleTime=-1  SaveFormat=Array
  To Workspace3 : ToWorkspace  VariableName=Phic  SampleTime=-1  SaveFormat=Array
  To Workspace4 : ToWorkspace  VariableName=T  SampleTime=-1  SaveFormat=Array
  UAV Weight : Constant  Value=mass  OutDataTypeMode=single
  UAV Pos1 : InportShadow  Port=1  SampleTime=apSampleTime  LatchByCopyingInsideSignal=off
  as_c to phi_c : SLUGS_Library/Navigation/as_c to phi_c  SystemSampleTime=-1
  phi_c : Outport
  h_c : Outport  Port=2
  wires:
  Compute WP Index/2(WP0) -> Get Wps Compute Frenet/1(WP Idx 0)
  Compute WP Index/3(WP1) -> Get Wps Compute Frenet/2(WP Idx 1)
  Get Wps Compute Frenet/2(N) -> Compute Lateral Error/1, "Park, Deyst & How Lat Accel Cmd"/3, To Workspace2/1
  Get Wps Compute Frenet/1(T) -> To Workspace4/1, Compute WP Index/1(T1), "Park, Deyst & How Lat Accel Cmd"/2
  Puav/1 -> Compute WP Index/2(Puav)
  Max WP Idx/1 -> Compute WP Index/3(Max WP Index)
  Start WP Idx/1 -> Compute WP Index/4(StartingWP)
  "Park, Deyst & How Lat Accel Cmd"/1 -> To Workspace1/1, as_c to phi_c/1
  UAV Pos1/1 -> Compute Lateral Error/3
  as_c to phi_c/1 -> phi_c/1, To Workspace3/1
  UAV Weight/1 -> as_c to phi_c/2
  Compute Lateral Error/1 -> "Park, Deyst & How Lat Accel Cmd"/4
  Get Wps Compute Frenet/3(WP 1) -> Compute Lateral Error/2, Selector/1, Compute WP Index/5("WP1 ")
  Selector/1 -> h_c/1
  L1 Base (m)/1 -> "Park, Deyst & How Lat Accel Cmd"/5
  Compute WP Index/1(WP Change) -> Get Wps Compute Frenet/Enable
  R/1 -> Compute WP Index/6(R)
  Vxyz/1 -> "Park, Deyst & How Lat Accel Cmd"/1
  WP Fly/1 -> Compute WP Index/7(WP Fly)
  Compute WP Index/4(UAV IC) -> Get Wps Compute Frenet/3(UAV IC)

== system SLUGS_Library/Navigation/Bank to Psi Dot ==
  phi_c : Inport
  U_m : Inport  Port=2
  Constant1 : Constant  Value=9.80665  OutDataTypeMode=single
  Divide : Product  Inputs=/*  OutDataTypeMode=single  OutScaling=2^-10
  Divide1 : Product  OutDataTypeMode=single  OutScaling=2^-10
  Subsystem8 : SLUGS_Library/Subsystem8  SystemSampleTime=-1
  negprotect : Stateflow chart
  psi_dot_c : Outport
  wires:
  U_m/1 -> negprotect/1(val)
  Constant1/1 -> Divide/2
  Divide1/1 -> psi_dot_c/1
  Subsystem8/1 -> Divide1/1
  phi_c/1 -> Subsystem8/1
  Divide/1 -> Divide1/2
  negprotect/1(zpVal) -> Divide/1

== system SLUGS_Library/Navigation/Compute Lateral Error ==
  N : Inport
  WP1 : Inport  Port=2
  UAV pos : Inport  Port=3
  Add : Sum  Inputs=+-  OutScaling=2^-10
  Subsystem3 : SLUGS_Library/Subsystem3  SystemSampleTime=-1
  Pe_lat : Outport
  wires:
  WP1/1 -> Add/1
  UAV pos/1 -> Add/2
  N/1 -> Subsystem3/1
  Add/1 -> Subsystem3/2
  Subsystem3/1 -> Pe_lat/1

== system SLUGS_Library/Navigation/Compute Distance ==
  Pos 1 : Inport
  Pos 2 : Inport  Port=2
  Add : Sum  Inputs=+-  OutScaling=2^-10
  Norm : SLUGS_Library/Navigation/Norm  SystemSampleTime=-1
  Dist : Outport
  wires:
  Pos 1/1 -> Add/1
  Pos 2/1 -> Add/2
  Add/1 -> Norm/1
  Norm/1 -> Dist/1

== system SLUGS_Library/Navigation/Compute Frenet ==
  Pos 1 : Inport
  Pos 2 : Inport  Port=2
  Add : Sum  Inputs=-+  OutScaling=2^-10
  Normalize Vector : SLUGS_Library/Navigation/Normalize Vector  SystemSampleTime=-1
  "Normalize Vector " : SLUGS_Library/Navigation/Normalize Vector  SystemSampleTime=-1
  Select N  Terms : Stateflow chart
  T : Outport
  N : Outport  Port=2
  wires:
  Pos 1/1 -> Add/1
  Pos 2/1 -> Add/2
  Add/1 -> Normalize Vector/1
  Normalize Vector/1 -> T/1, Select N  Terms/1(T)
  Select N  Terms/1(N) -> "Normalize Vector "/1
  "Normalize Vector "/1 -> N/1

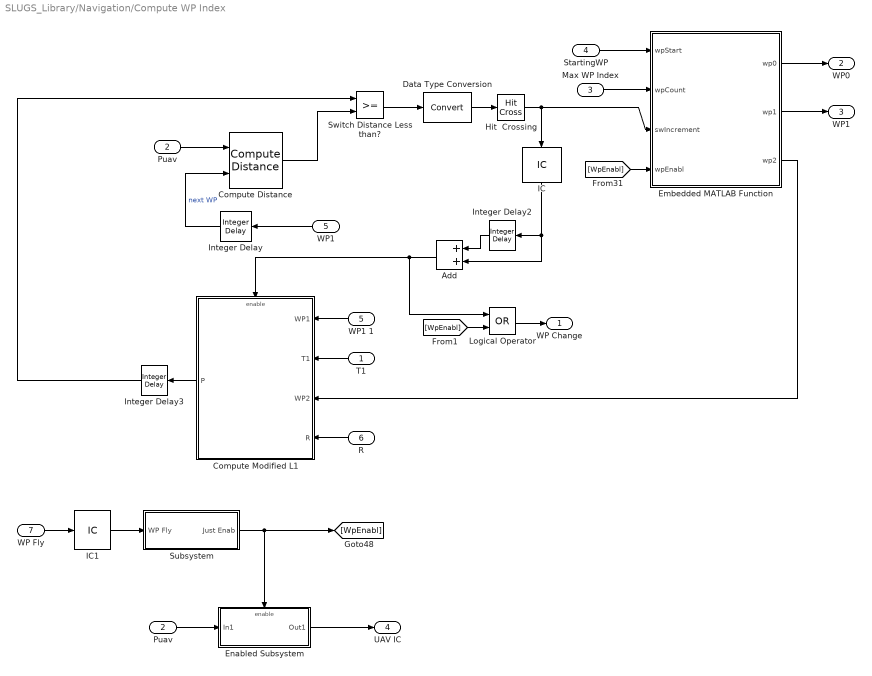
== system SLUGS_Library/Navigation/Compute WP Index ==
  T1 : Inport  Orientation=left
  Puav : Inport  Port=2
  Max WP Index : Inport  Port=3
  StartingWP : Inport  Port=4
  "WP1 " : Inport  Orientation=left  Port=5
  R : Inport  Orientation=left  Port=6
  WP Fly : Inport  Port=7
  Add : Sum  Orientation=left  Inputs=2  OutScaling=2^-10
  Compute Distance : SLUGS_Library/Navigation/Compute Distance  SystemSampleTime=-1
  Compute Modified L1 : Subsystem  Orientation=left
  Data Type Conversion : DataTypeConversion  OutDataTypeMode=double  SampleTime=apSampleTime
  Embedded MATLAB Function : Stateflow chart
  Enabled Subsystem : Subsystem  TreatAsAtomicUnit=on
  Hit  Crossing : HitCross  HitCrossingOffset=0.9  HitCrossingDirection=rising  SampleTime=apSampleTime
  IC : InitialCondition  Orientation=down
  IC1 : InitialCondition  Value=0
  Integer Delay : simulink/Discrete/Integer Delay  Orientation=left  vinit=0.0  samptime=-1  NumDelays=1
  Integer Delay2 : simulink/Discrete/Integer Delay  Orientation=left  vinit=0  samptime=-1  NumDelays=1
  Integer Delay3 : simulink/Discrete/Integer Delay  Orientation=left  vinit=150  samptime=-1  NumDelays=1
  Logical Operator : Logic  Operator=OR  AllPortsSameDT=off  OutDataTypeMode=Boolean
  "Puav " : InportShadow  Port=2  LatchByCopyingInsideSignal=off
  Subsystem : Subsystem
  Switch Distance Less than? : RelationalOperator  LogicOutDataTypeMode=Boolean  LogicDataType=double()  SampleTime=apSampleTime
  WP1 1 : InportShadow  Orientation=left  Port=5  LatchByCopyingInsideSignal=off
  WP Change : Outport
  WP0 : Outport  Port=2
  WP1 : Outport  Port=3
  UAV IC : Outport  Port=4
  wires:
  Integer Delay/1 -> Compute Distance/2  "next WP"
  Puav/1 -> Compute Distance/1
  Embedded MATLAB Function/2(wp1) -> WP1/1
  Embedded MATLAB Function/1(wp0) -> WP0/1
  StartingWP/1 -> Embedded MATLAB Function/1(wpStart)
  Switch Distance Less than?/1 -> Data Type Conversion/1
  Max WP Index/1 -> Embedded MATLAB Function/2(wpCount)
  Compute Distance/1 -> Switch Distance Less than?/2
  "WP1 "/1 -> Integer Delay/1
  Hit  Crossing/1 -> Embedded MATLAB Function/3(swIncrement), IC/1
  Data Type Conversion/1 -> Hit  Crossing/1
  Embedded MATLAB Function/3(wp2) -> Compute Modified L1/3(WP2)
  WP1 1/1 -> Compute Modified L1/1(WP1)
  T1/1 -> Compute Modified L1/2(T1)
  Integer Delay2/1 -> Add/1
  Add/1 -> Compute Modified L1/Enable, Logical Operator/1
  IC/1 -> Add/2, Integer Delay2/1
  Compute Modified L1/1(P) -> Integer Delay3/1
  Integer Delay3/1 -> Switch Distance Less than?/1
  R/1 -> Compute Modified L1/4(R)
  WP Fly/1 -> IC1/1
  Subsystem/1(Just Enab) -> Enabled Subsystem/Enable, [WpEnabl]
  "Puav "/1 -> Enabled Subsystem/1(In1)
  Enabled Subsystem/1(Out1) -> UAV IC/1
  IC1/1 -> Subsystem/1(WP Fly)
  [WpEnabl] -> Embedded MATLAB Function/4(wpEnabl)
  Logical Operator/1 -> WP Change/1
  [WpEnabl] -> Logical Operator/2

== system SLUGS_Library/Navigation/Norm ==
  Vector : Inport
  Subsystem1 : SLUGS_Library/Subsystem1  SystemSampleTime=-1
  Subsystem3 : SLUGS_Library/Subsystem3  SystemSampleTime=-1
  Norm : Outport
  wires:
  Subsystem3/1 -> Subsystem1/1
  Vector/1 -> Subsystem3/2, Subsystem3/1
  Subsystem1/1 -> Norm/1

== system SLUGS_Library/Navigation/Normalize Vector ==
  Vector : Inport
  Divide : Product  Inputs=*/  OutScaling=2^-10
  Norm : SLUGS_Library/Navigation/Norm  SystemSampleTime=-1
  Zero Bound : Saturate  UpperLimit=inf  LowerLimit=0.001
  Normalized : Outport
  wires:
  Divide/1 -> Normalized/1
  Zero Bound/1 -> Divide/2
  Norm/1 -> Zero Bound/1
  Vector/1 -> Divide/1, Norm/1

== system SLUGS_Library/Navigation/Park, Deyst & How Lat Accel Cmd ==
  Vxyz : Inport
  T : Inport  Port=2
  N : Inport  Port=3
  Pe_lat : Inport  Port=4
  L1 : Inport  Port=5
  Compute Eta : Subsystem
  Compute L1 Vector LINE MODE : Subsystem
  "L1 " : InportShadow  Port=5  LatchByCopyingInsideSignal=off
  Park's Lateral Accel Command : Subsystem
  a_s_c : Outport
  wires:
  Park's Lateral Accel Command/1(a_s_c) -> a_s_c/1
  Compute L1 Vector LINE MODE/1(L1_vec) -> Compute Eta/2(L1_vec)
  Compute Eta/1(Eta) -> Park's Lateral Accel Command/3(eta)
  Vxyz/1 -> Compute Eta/1(Vxyz), Park's Lateral Accel Command/1(Vxyz)
  "L1 "/1 -> Park's Lateral Accel Command/2(L1)
  Pe_lat/1 -> Compute L1 Vector LINE MODE/1(Pe_lat)
  L1/1 -> Compute L1 Vector LINE MODE/2(L1)
  T/1 -> Compute L1 Vector LINE MODE/3(T)
  N/1 -> Compute L1 Vector LINE MODE/4(N)

== system SLUGS_Library/Navigation/as_c to phi_c ==
  as_c : Inport
  W : Inport  Port=2
  Divide : Product  Inputs=*/  OutScaling=2^-10
  Subsystem2 : SLUGS_Library/Subsystem2  SystemSampleTime=-1
  phi_c : Outport
  wires:
  Divide/1 -> Subsystem2/1
  as_c/1 -> Divide/1
  Subsystem2/1 -> phi_c/1
  W/1 -> Divide/2

== system SLUGS_Library/Navigation/get WP Coord from Index ==
  WP Idx : Inport
  C Function Call : dsPICdrivers/OTHERS/C Function Call  Tag=dsPIC_dsPIC_CFunctionCall  fctName='getWP'  INPUT_SIZE=1  INPUT1=uint8  INPUT2=--  INPUT3=--  OUTPUT_SIZE=3  OUTPUT1=real32  SampleTime=-1  InputType=[ 2 ]  OutputType=[ 7 ]  FctDeclaration=extern void getWP(uint8_T u1,real32_T* y1);  FctCall=getWP(%u1, *%y1);  OrderingInOutPopup=None
  Data Type Conversion : DataTypeConversion  OutDataTypeMode=double
  Data Type Conversion1 : DataTypeConversion  OutDataTypeMode=single
  Environment Controller : simulink/Signal Routing/Environment Controller  SystemSampleTime=-1
  MATLAB Fcn : MATLABFcn  MATLABFcn=Xpoints(u(1))  OutputDimensions=1  OutputSignalType=real
  MATLAB Fcn1 : MATLABFcn  MATLABFcn=Ypoints(u(1))  OutputDimensions=1
  MATLAB Fcn2 : MATLABFcn  MATLABFcn=Zpoints(u(1))  OutputDimensions=1
  Mux : Mux  Inputs=3
  WP Coord : Outport
  wires:
  Data Type Conversion1/1 -> Environment Controller/1
  Data Type Conversion/1 -> MATLAB Fcn2/1, MATLAB Fcn/1, MATLAB Fcn1/1
  MATLAB Fcn/1 -> Mux/1
  MATLAB Fcn1/1 -> Mux/2
  MATLAB Fcn2/1 -> Mux/3
  WP Idx/1 -> Data Type Conversion/1, C Function Call/1
  Mux/1 -> Data Type Conversion1/1
  Environment Controller/1 -> WP Coord/1
  C Function Call/1 -> Environment Controller/2

== system SLUGS_Library/Navigation/psi_dot to Bank ==
  psi_dot_c : Inport
  U_m : Inport  Port=2
  Constant1 : Constant  Value=9.80665  OutDataTypeMode=single
  Divide : Product  Inputs=**/  OutScaling=2^-10
  Subsystem2 : SLUGS_Library/Subsystem2  SystemSampleTime=-1
  phi_c : Outport
  wires:
  psi_dot_c/1 -> Divide/1
  U_m/1 -> Divide/2
  Constant1/1 -> Divide/3
  Subsystem2/1 -> phi_c/1
  Divide/1 -> Subsystem2/1
